simulink model "motor"  (R2025b)
settings: Solver=VariableStepAuto  StartTime=0.0  StopTime=1000  RelTol=1e-3
settings Model: Creator=airat  LastModifiedBy=airat

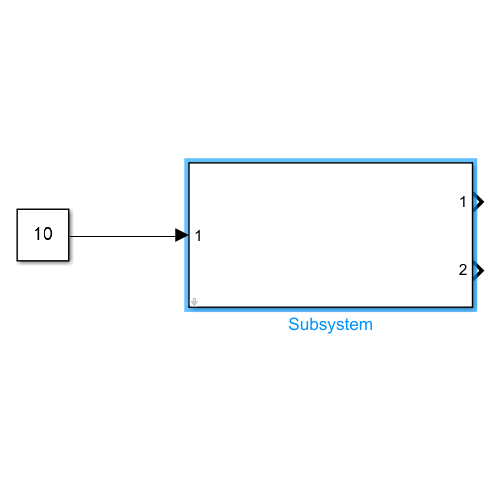
[thumbnail: Simulink's stored preview of the top-level diagram]
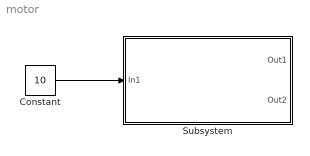
== system motor ==
  Constant : Constant  Value=10
  Subsystem : Subsystem  mask{Lov=0.013, Lr=0.0015, Rr=8, Cw=3.15, Cm=1.3, Y=7*10^(-6)}
  wires:
  Constant/1 -> Subsystem/1(In1)

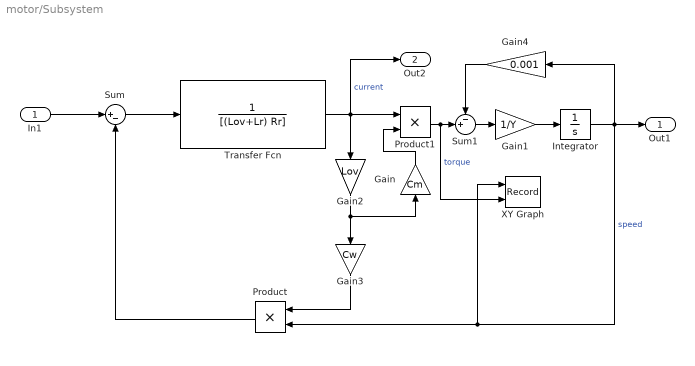
== system motor/Subsystem ==
  In1 : Inport
  Gain : Gain  Gain=Cm
  Gain1 : Gain  Gain=1/Y
  Gain2 : Gain  Gain=Lov
  Gain3 : Gain  Gain=Cw
  Gain4 : Gain  Gain=0.001
  Integrator : Integrator
  Product : Product
  Product1 : Product
  Sum : Sum  Inputs=|+-
  Sum1 : Sum  Inputs=-+|
  Transfer Fcn : TransferFcn  Denominator=[(Lov+Lr) Rr]
  XY Graph : Record  NumPorts=2.0  FileSettingsInternal="{\"entries\":[{\"content\":{\"excelSettings\":{\"content\":{},\"type\":\"Streamout.ExcelSettings\"},\"parquetSettings\":{\"content\":{},\"type\":\"Streamout.ParquetSettings\"}},\"type\":\"Streamout.FileSettingStorage\",\"uuid\":\"\"}],\"packageUris\":[\"http:\\/\\/schema.mathworks.com\\/mf0\\/streamout_blocks\\/R2020a\"],\"version\":\"1.0\"}"  FrameSettings=[0, 0]  Layout=[1 1]  SignalsInternal="{\"entries\":[{\"content\":{\"signals\":[{\"content\":{\"blockPath\":[],\"dimensions\":[1],\"domain\":\"\",\"lineColor\":\"#a2142f\",\"plots\":[ 1 ],\"port\":1,\"sid\":[\"\"],\"signalID\":1,\"signalName\":\"speed\"},\"type\":\"RecordBlkView.Signal\",\"uuid\":\"\"},{\"content\":{\"blockPath\":[],\"dimensions\":[1],\"domain\":\"\",\"lineColor\":\"#139fff\",\"plots\":[ 1 ],\"port\":2,\"sid\":[\"\"],\"signalID\":2,\"signalName\":\"torque\"},\"type\":\"RecordBlkView.Signal\",\"uuid\":\"\"}]},\"type\":\"RecordBlkView.InputSignals\",\"uuid\":\"\"}],\"packageUris\":[\"http:\\/\\/schema.mathworks.com\\/mf0\\/streamout_blocks\\/R2020a\"],\"version\":\"1.0\"}"  VisualizationBindings="{\"xyplotplugin\":{\"info\":[{\"series\":[{\"bindingParametersList\":[{\"parameter\":\"X-Axis\",\"signalID\":2,\"signalName\":\"torque\"},{\"parameter\":\"Y-Axis\",\"signalID\":1,\"signalName\":\"speed\"},{\"parameter\":\"X-Axis\",\"signalID\":2,\"signalName\":\"torque\"},{\"parameter\":\"Y-Axis\",\"signalID\":1,\"signalName\":\"speed\"}],\"seriesID\":0}],\"subplotID\":1}]}}"  CompatibilityTag=XY
  Out1 : Outport
  Out2 : Outport  Port=2
  wires:
  Sum/1 -> Transfer Fcn/1
  In1/1 -> Sum/1
  Transfer Fcn/1 -> Out2/1, Product1/1, Gain2/1  "current"
  Gain1/1 -> Integrator/1
  Integrator/1 -> Gain4/1, Out1/1, XY Graph/1, Product/2  "speed"
  Gain2/1 -> Gain/1, Gain3/1
  Gain3/1 -> Product/1
  Product/1 -> Sum/2
  Gain/1 -> Product1/2
  Product1/1 -> XY Graph/2, Sum1/2  "torque"
  Sum1/1 -> Gain1/1
  Gain4/1 -> Sum1/1
